simulink model "KinematicsIntegration"  (R2018a)
settings: Solver=VariableStepAuto  StartTime=0.0  StopTime=10.0  RelTol=1e-3
PreLoadFcn:
  | modelDir = fileparts(get_param(bdroot, 'FileName'));
  | addpath(fullfile(modelDir,'../../Parameters'));
  | addpath(fullfile(modelDir,'../../Model/generated'));
  | 
  | Constants_Kugle
  | Constants_nominal
  | Parameters_General
  | Parameters_Controllers
InitFcn:
  | Constants_Kugle
  | Constants_nominal
  | Parameters_General
  | Parameters_Controllers
undefined symbols (not defined in the file or in its folder): constants_nominal, DiscIntNeverNeededParam, TicksPrRev, Ts, x_init
libraries: simulink x1
settings Model: Creator=Thomas  LastModifiedBy=Thomas

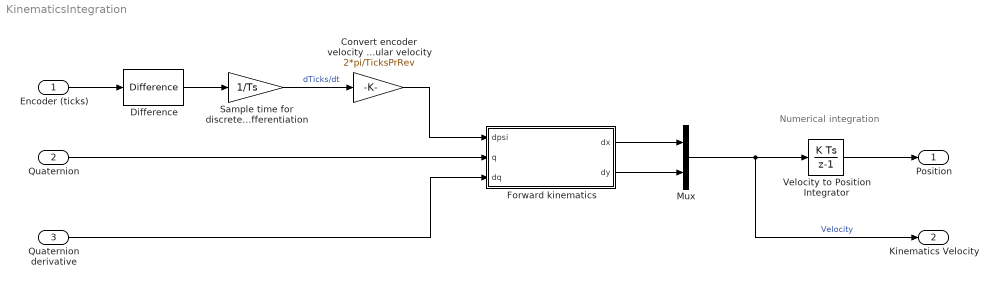
== system KinematicsIntegration ==
  note: Numerical integration
  Encoder (ticks) : Inport  PortDimensions=3
  Quaternion : Inport  Port=2
  Quaternion derivative : Inport  Port=3
  Convert encoder velocity to angular velocity : Gain  Gain=2*pi/TicksPrRev
  "Difference " : simulink/Discrete/Difference  ICPrevInput=0.0  OutMin=[]  OutMax=[]  OutDataType=fixdt(1, 16)  OutScaling=2^-10  DoSatur=off
  Forward kinematics : Subsystem
  Mux : Mux  Inputs=2
  Sample time for discrete differentiation : Gain  Gain=1/Ts
  Velocity to Position Integrator : DiscreteIntegrator  InitialCondition=x_init(1:2)  SampleTime=Ts  ICPrevOutput=DiscIntNeverNeededParam  ICPrevScaledInput=DiscIntNeverNeededParam
  Position : Outport
  Kinematics Velocity : Outport  Port=2
  wires:
  Forward kinematics/2(dy) -> Mux/2
  Mux/1 -> Kinematics Velocity/1, Velocity to Position Integrator/1  "Velocity"
  Forward kinematics/1(dx) -> Mux/1
  Encoder (ticks)/1 -> "Difference "/1
  Sample time for discrete differentiation/1 -> Convert encoder velocity to angular velocity/1  "dTicks/dt"
  "Difference "/1 -> Sample time for discrete differentiation/1
  Convert encoder velocity to angular velocity/1 -> Forward kinematics/1(dpsi)
  Velocity to Position Integrator/1 -> Position/1
  Quaternion/1 -> Forward kinematics/2(q)
  Quaternion derivative/1 -> Forward kinematics/3(dq)

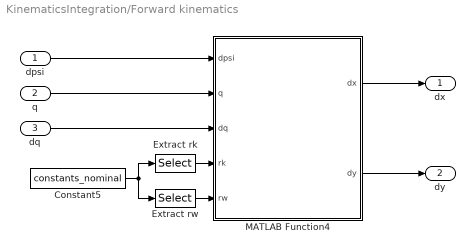
== system KinematicsIntegration/Forward kinematics ==
  dpsi : Inport
  q : Inport  Port=2
  dq : Inport  Port=3
  Constant5 : Constant  Value=constants_nominal
  Extract rk : Selector  InputPortWidth=13  IndexOptions=Index vector (dialog)  Indices=[3]  OutputSizes=1
  Extract rw : Selector  InputPortWidth=13  IndexOptions=Index vector (dialog)  Indices=[9]  OutputSizes=1
  MATLAB Function4 : MATLAB Function  TreatAsAtomicUnit=on
  dx : Outport
  dy : Outport  Port=2
  wires:
  q/1 -> MATLAB Function4/2(q)
  MATLAB Function4/1(dx) -> dx/1
  dpsi/1 -> MATLAB Function4/1(dpsi)
  MATLAB Function4/2(dy) -> dy/1
  dq/1 -> MATLAB Function4/3(dq)
  Extract rk/1 -> MATLAB Function4/4(rk)
  Extract rw/1 -> MATLAB Function4/5(rw)
  Constant5/1 -> Extract rw/1, Extract rk/1

== matlab function KinematicsIntegration/Forward kinematics/MATLAB Function4 ==
  data: dpsi input size=3; dx output size=1; q input size=4; dq input size=4; rk input; rw input; dy output size=1
function [dx, dy] = ForwardKinematics(dpsi,q,dq,rk,rw)

q1 = q(1);
q2 = q(2);
q3 = q(3);
q4 = q(4);

dq1 = dq(1);
dq2 = dq(2);
dq3 = dq(3);
dq4 = dq(4);

dpsi1 = dpsi(1);
dpsi2 = dpsi(2);
dpsi3 = dpsi(3);

dxdy = ForwardKinematics(dpsi1,dpsi2,dpsi3,dq1,dq2,dq3,dq4,q1,q2,q3,q4,rk,rw);

dx = dxdy(1);
dy = dxdy(2);
